simulink model "MWT_model"  (R2021b)
settings: Solver=VariableStepAuto  StartTime=0.0  StopTime=600  RelTol=1e-3
values from neighbouring files (symbols this model uses):
  Bt = 1e-6    (= 1e-06)    [MWT_model_input.m]
  Jt = 13.6e-7+1e-4    (= 0.00010136)    [MWT_model_input.m]
  Ke = Kt    (= 0.0139)    [MWT_model_input.m]
  Kt = 13.9e-3    (= 0.0139)    [MWT_model_input.m]
  La = 0.227    [MWT_model_input.m]
  p = 1.225    [MWT_model_input.m]
  p00 = 0.06736    [MWT_model_input.m]
  p01 = 0.279    [MWT_model_input.m]
  p02 = -0.09197    [MWT_model_input.m]
  p03 = 0.006537    [MWT_model_input.m]
  p10 = -0.01231    [MWT_model_input.m]
  p11 = 0.003341    [MWT_model_input.m]
  p12 = 0.002017    [MWT_model_input.m]
  p13 = -0.0001495    [MWT_model_input.m]
  p20 = 0.0001297    [MWT_model_input.m]
  p21 = -3.639e-05    [MWT_model_input.m]
  p22 = -1.063e-06    [MWT_model_input.m]
  p23 = 2.226e-07    [MWT_model_input.m]
  p30 = -4.46e-07    [MWT_model_input.m]
  p31 = 7.744e-08    [MWT_model_input.m]
  p32 = -1.905e-09    [MWT_model_input.m]
  p40 = 6.032e-10    [MWT_model_input.m]
  p41 = -4.972e-11    [MWT_model_input.m]
  p50 = -2.734e-13    [MWT_model_input.m]
  R = 0.75    [MWT_model_input.m]
  Ra = 2.07    [MWT_model_input.m]
  Vm = 3    [MWT_model_input.m]
  wcmax = 700    [MWT_model_input.m]
undefined symbols (not defined in the file or in its folder): sigbuilder_block
libraries: RCTblocks x2, simulink x1, slpidlib x1, autolibsharedcoupling x1
settings Model: Creator=alevl  LastModifiedBy=alevl

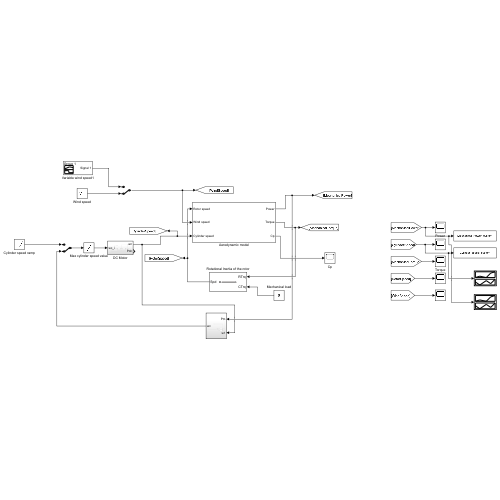
[thumbnail: Simulink's stored preview of the top-level diagram]
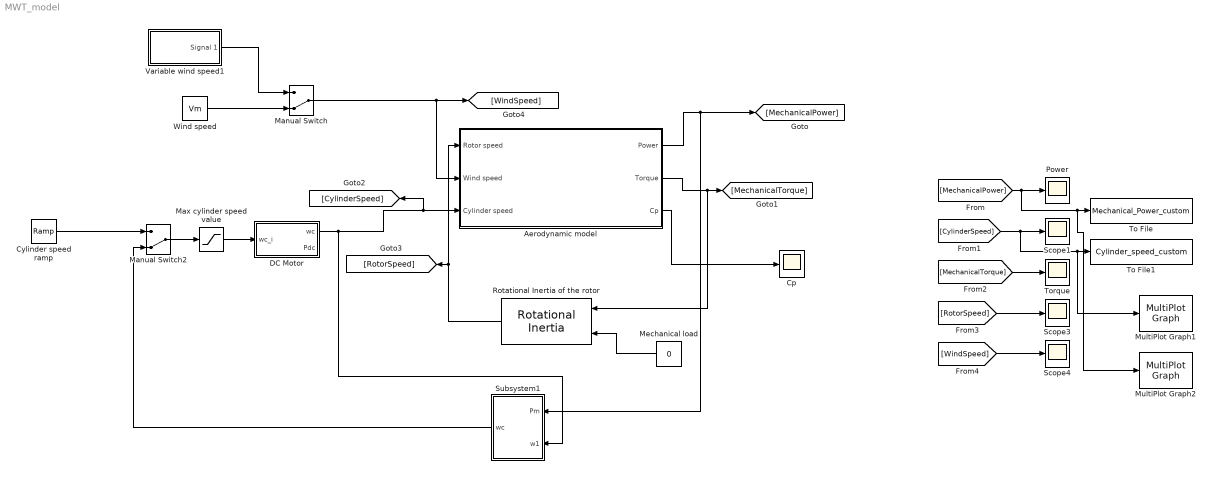
== system MWT_model ==
  Aerodynamic model : Subsystem
  Cp : Scope
  Cylinder speed ramp : simulink/Sources/Ramp  slope=1  start=0  InitialOutput=0
  DC Motor : Subsystem
  Manual Switch : ManualSwitch  CurrentSetting=0
  Manual Switch2 : ManualSwitch  CurrentSetting=0
  Max cylinder speed value : Saturate  UpperLimit=wcmax
  Mechanical load : Constant  Value=0
  MultiPlot Graph1 : RCTblocks/MultiPlot Graph  Tag=MultiPlot  tmin=0  tmax=350  ymin=0  ymax=700  Tsamp=-1  vnamesave=multisimout1
      settings: SourceProductBaseCode=RC
  MultiPlot Graph2 : RCTblocks/MultiPlot Graph  Tag=MultiPlot  tmin=0  tmax=350  ymin=0  ymax=600  Tsamp=-1  vnamesave=multisimout2
      settings: SourceProductBaseCode=RC
  Power : Scope
  Rotational Inertia of the rotor : autolibsharedcoupling/Rotational Inertia  port_config=Simulink  extInfo=off  externJ=off  J=2  b=1.4  omega_o=0.001  blkID=0  aMode=2
      settings: SourceProductBaseCode=PW,DR,MT,UV,VE
  Scope1 : Scope
  Scope3 : Scope
  Scope4 : Scope
  Subsystem1 : Subsystem
  To File : ToFile  Filename=Mechanical_Power_custom  MatrixName=P_NMPPT  SampleTime=0.01
  To File1 : ToFile  Filename=Cylinder_speed_custom  MatrixName=W_NMPPT  SampleTime=0.01
  Torque : Scope
  Variable wind speed1 : Subsystem  Tag=STV Subsys  LoadFcn=sigbuilder_block('load');  StartFcn=sigbuilder_block('start');  StopFcn=sigbuilder_block('stop');  ClipboardFcn=sigbuilder_block('clipboard');  mask(Sigbuilder block){tuvar=[0:10]}
      mask help: Simulink:masks:SigbuilderBlock_MD
      mask init:
      | if ~strcmp(get_param(bdroot(gcbh),'SimulationStatus'),'stopped') tuvar = sigbuilder_block('maskInit'); end
      settings: CopyFcn=sigbuilder_block('copy');  DeleteFcn=sigbuilder_block('delete');  ModelCloseFcn=sigbuilder_block('modelClose');  PreSaveFcn=sigbuilder_block('preSave');  PauseFcn=sigbuilder_block('pause');  ContinueFcn=sigbuilder_block('continue');  NameChangeFcn=sigbuilder_block('namechange');  OpenFcn=sigbuilder_block('open',[5.4 5.4 1141.2 580.8 ]);  CloseFcn=sigbuilder_block('close');
      mask Display: plot(0, 0, 100, 100,[2, 2, 32, 32, 2], [68, 8, 8, 68, 68],[32, 2], [38, 38], [32, 19, 2],[53, 60, 44], [32, 17, 17, 2],[16, 16, 31, 31]);txt = getActiveGroup(gcbh);text(2, 100, txt,'verticalAlignment', 'top');
  Wind speed : Constant  Value=Vm
  wires:
  Aerodynamic model/2(Torque) -> Rotational Inertia of the rotor/1, [MechanicalTorque]
  Rotational Inertia of the rotor/1 -> [RotorSpeed], Aerodynamic model/1(Rotor speed)
  Wind speed/1 -> Manual Switch/2
  Variable wind speed1/1(Signal 1) -> Manual Switch/1
  Manual Switch/1 -> Aerodynamic model/2(Wind speed), [WindSpeed]
  Cylinder speed ramp/1 -> Manual Switch2/1
  [MechanicalPower] -> MultiPlot Graph2/1, To File/1, Power/1
  [CylinderSpeed] -> MultiPlot Graph1/1, To File1/1, Scope1/1
  [MechanicalTorque] -> Torque/1
  [RotorSpeed] -> Scope3/1
  [WindSpeed] -> Scope4/1
  Aerodynamic model/1(Power) -> Subsystem1/1(Pm), [MechanicalPower]
  Aerodynamic model/3(Cp) -> Cp/1
  Mechanical load/1 -> Rotational Inertia of the rotor/2
  Manual Switch2/1 -> Max cylinder speed value/1
  Max cylinder speed value/1 -> DC Motor/1(wc_i)
  DC Motor/1(wc) -> Subsystem1/2(w1), Aerodynamic model/3(Cylinder speed), [CylinderSpeed]
  Subsystem1/1(wc) -> Manual Switch2/2

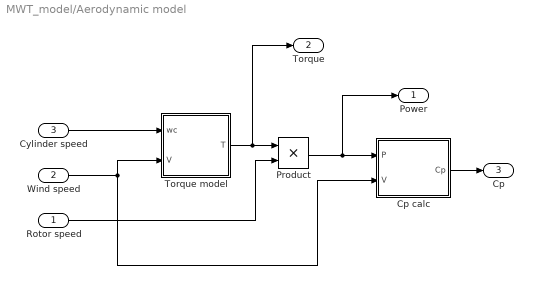
== system MWT_model/Aerodynamic model ==
  Rotor speed : Inport
  Wind speed : Inport  Port=2
  Cylinder speed : Inport  Port=3
  Cp calc : MATLAB Function  TreatAsAtomicUnit=on
  Product : Product
  Torque model : MATLAB Function  TreatAsAtomicUnit=on
  Power : Outport
  Torque : Outport  Port=2
  Cp : Outport  Port=3
  wires:
  Cylinder speed/1 -> Torque model/1(wc)
  Wind speed/1 -> Cp calc/2(V), Torque model/2(V)
  Torque model/1(T) -> Torque/1, Product/1
  Rotor speed/1 -> Product/2
  Product/1 -> Power/1, Cp calc/1(P)
  Cp calc/1(Cp) -> Cp/1

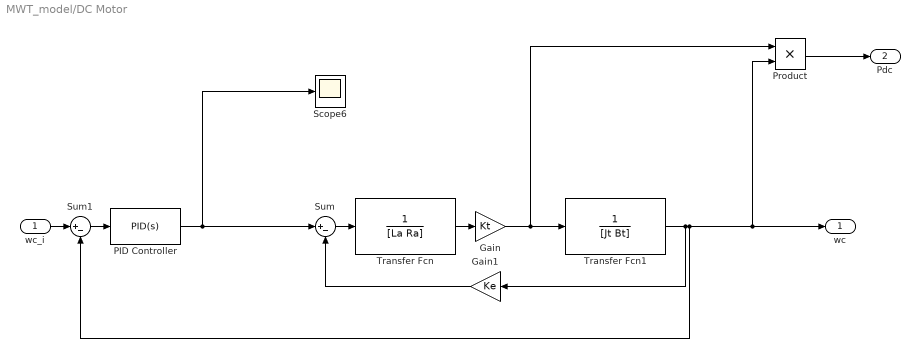
== system MWT_model/DC Motor ==
  wc_i : Inport
  Gain : Gain  Gain=Kt
  Gain1 : Gain  Gain=Ke
  PID Controller : slpidlib/PID Controller  Controller=PID  Form=Parallel  TimeDomain=Continuous-time  UseExternalTs=off  SampleTime=-1  IntegratorMethod=Forward Euler  FilterMethod=Forward Euler  ControllerParametersSource=internal  P=0.272229131767828  I=0.561292736049152  D=0.0312749136462088  UseFilter=on  N=2096.81611582006  TunerSelectOption=Transfer Function Based (PID Tuner App)  InitialConditionSource=internal  InitialConditionForIntegrator=0  InitialConditionForFilter=0  DifferentiatorICPrevScaledInput=0  ExternalReset=none  TrackingMode=off  Kt=1  LimitOutput=on  SatLimitsSource=internal  UpperSaturationLimit=12  LowerSaturationLimit=-12  LinearizeAsGain=on  AntiWindupMode=none  Kb=1  POutMin=[]  POutMax=[]  IOutMin=[]  IOutMax=[]  DOutMin=[]  DOutMax=[]  NOutMin=[]  NOutMax=[]  SumOutMin=[]  SumOutMax=[]  SaturationOutMin=[]  SaturationOutMax=[]  PParamMin=[]  PParamMax=[]  IParamMin=[]  IParamMax=[]  DParamMin=[]  DParamMax=[]  NParamMin=[]  NParamMax=[]  KbParamMin=[]  KbParamMax=[]  KtParamMin=[]  KtParamMax=[]  KbOutMin=[]  KbOutMax=[]  KtOutMin=[]  KtOutMax=[]  IntegratorOutMin=[]  IntegratorOutMax=[]  FilterOutMin=[]  FilterOutMax=[]  SumI1OutMin=[]  SumI1OutMax=[]  SumI2OutMin=[]  SumI2OutMax=[]  SumI3OutMin=[]  SumI3OutMax=[]  SumI4OutMin=[]  SumI4OutMax=[]  SumDOutMin=[]  SumDOutMax=[]  DifferentiatorOutMin=[]  DifferentiatorOutMax=[]  FilterDiffOutCoefMin=[]  FilterDiffOutCoefMax=[]  ReciprocalOutMin=[]  ReciprocalOutMax=[]  SumDenOutMin=[]  SumDenOutMax=[]  SumNumOutMin=[]  SumNumOutMax=[]  DivideOutMin=[]  DivideOutMax=[]  UdiffTsProdOutMin=[]  UdiffTsProdOutMax=[]  NTsProdOutMin=[]  NTsProdOutMax=[]  UintegralTsProdOutMin=[]  UintegralTsProdOutMax=[]  UngainTsProdOutMin=[]  UngainTsProdOutMax=[]  IntegratorContinuousStateAttributes=''  IntegratorStateMustResolveToSignalObject=off  IntegratorRTWStateStorageClass=Auto  FilterContinuousStateAttributes=''  FilterStateMustResolveToSignalObject=off  FilterRTWStateStorageClass=Auto  ParallelPVariant=InternalParameters  IdealPVariant=Disabled  IVariant=InternalParameters  DVariant=InternalParameters  IntegratorVariant=Continuous  SatVariant=Enabled  AWVariant=Passthrough  PCopyVariant=Disabled  TRVariant=Disabled  FdbkBlocksVariant=Forward  IdealPFdbkVariant=Disabled  SatFdbkVariant=Disabled  DerivativeFilterVariant=ContFilter  NVariant=InternalParameters  NCopyVariant=Disabled  FilterICVariant=InternalICsFilter  IntegratorICVariant=InternalICs  ExternalResetVariant=Disabled  TRSumVariant=Passthrough  SumFdbkVariant=Disabled  SumVariant=Sum_PID  TsampFilterVariant=InternalTs  TsampNgainVariant=Passthrough  TsampIntegralVariant=Passthrough  ExternalSaturationOutDataTypeStr=Inherit: Same as second input
  Product : Product
  Scope6 : Scope
  Sum : Sum  Inputs=|+-
  Sum1 : Sum  Inputs=|+-
  Transfer Fcn : TransferFcn  Denominator=[La Ra]
  Transfer Fcn1 : TransferFcn  Denominator=[Jt Bt]
  wc : Outport
  Pdc : Outport  Port=2
  wires:
  Transfer Fcn1/1 -> Product/2, wc/1, Sum1/2, Gain1/1
  wc_i/1 -> Sum1/1
  Sum1/1 -> PID Controller/1
  Gain1/1 -> Sum/2
  Sum/1 -> Transfer Fcn/1
  Product/1 -> Pdc/1
  Transfer Fcn/1 -> Gain/1
  PID Controller/1 -> Sum/1, Scope6/1
  Gain/1 -> Product/1, Transfer Fcn1/1

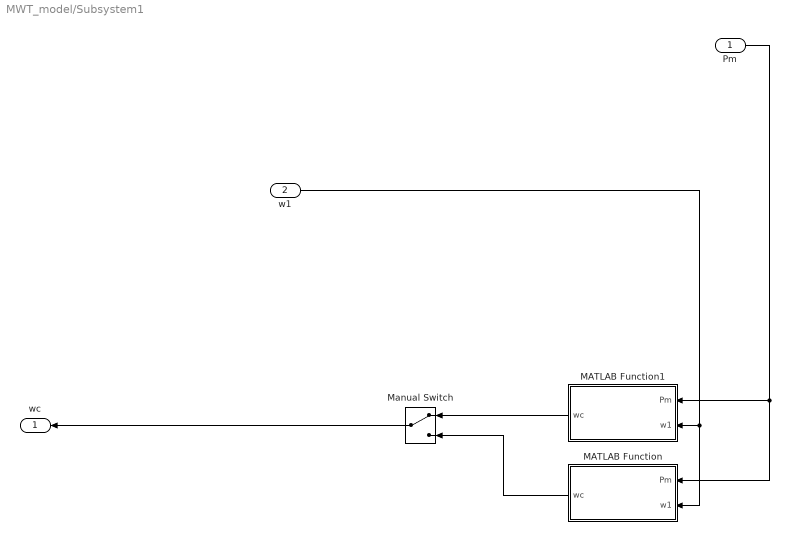
== system MWT_model/Subsystem1 ==
  Pm : Inport
  w1 : Inport  Port=2
  MATLAB Function : MATLAB Function  TreatAsAtomicUnit=on  SystemSampleTime=1
  MATLAB Function1 : MATLAB Function  TreatAsAtomicUnit=on  SystemSampleTime=1
  Manual Switch : ManualSwitch
  wc : Outport
  wires:
  MATLAB Function/1(wc) -> Manual Switch/2
  Pm/1 -> MATLAB Function/1(Pm), MATLAB Function1/1(Pm)
  w1/1 -> MATLAB Function/2(w1), MATLAB Function1/2(w1)
  MATLAB Function1/1(wc) -> Manual Switch/1
  Manual Switch/1 -> wc/1

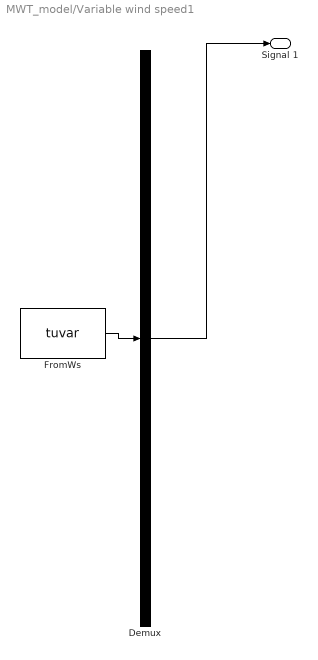
== system MWT_model/Variable wind speed1 ==
  Demux : Demux  Tag=STV Demux  Outputs=1
      settings: DisplayOption=none
  FromWs : FromWorkspace  Tag=STV FromWs  VariableName=tuvar
      SigBuilderData=|
      | common.afterFinalStr = 'Extrapolate'
      | common.sampleTime = 0
      | dataSet.timeRange = [0 350]
      | dataSet.name = 'Group 1'
      | sbobj.Groups.Name = 'Group 1'
      | sbobj.Groups.Signals.Name = 'Signal 1'
      | sbobj.Groups.Signals.XData = [0 50 50 100 100 150 150 200 200 250 250 300 300 350]
      | sbobj.Groups.Signals.YData = [2.5 2.5 5 5 7.5 7.5 10 10 7.5 7.5 5 5 2.5 2.5]
      | sbobj.Groups.TimeRange = [0 350]
  Signal 1 : Outport  Tag=STV Outport
  wires:
  FromWs/1 -> Demux/1
  Demux/1 -> Signal 1/1

== matlab function MWT_model/Subsystem1/MATLAB Function ==
  data: Pm input; wc output; w1 input
function wc = MPPT(Pm,w1)

%задание величин скорости вращения и мощности последовательными
persistent Pold wcold

%Задание начальных значений скорости вращения и мощности на первом шаге
if isempty (wcold)
    Pold=0;
    wcold=0;
end

%задание параметров алгоритма
wstep=30;

%цикл увеличения/уменьшения параметра исходя из состояния системы
if (Pm-Pold)>=0
    if (w1-wcold)>=0
        wc=w1+wstep;
    else
        wc=w1-wstep;
    end
else
    if (w1-wcold)>=0
        wc=w1-wstep;
    else
        wc=w1+wstep;
    end
end
%обвновление значений параметров по окончании цикла
wcold=w1;
Pold=Pm;

== matlab function MWT_model/Subsystem1/MATLAB Function1 ==
  data: Pm input; wc output; w1 input
function wc = HS_MPPT(Pm,w1)

%задание величин скорости вращения и мощности последовательными
persistent Pold wcold wstep i j EP
%Задание начальных значений скорости вращения и мощности на первом шаге
if isempty (wcold)
    Pold=0;
    wcold=0;
    wstep=30;
    i=0;
    j=0;
    EP=0;
end

%задание параметров алгоритма

EP=abs((Pold-Pm)/Pold)*100;
%цикл увеличения/уменьшения параметра исходя из состояния системы

if (Pm-Pold)>=0
    if (w1-wcold)>=0
        wc=w1+wstep;
    else
        wc=w1-wstep;
    end
else
    if (w1-wcold)>=0
        wc=w1-wstep;
    else
        wc=w1+wstep;
        wstep=wstep/2;
    end
end

% if (EP>0)&&(EP<=0.1)
%     wc=w1;
%     i=i+1;
% end

% if (i>2)&&(EP>0.1)
%     wstep=30;
%     i=0;
% end

if (EP>5)
    wstep=30;
    i=0;
end




if (wstep>30)
    wstep=30;
end


%обвновление значений параметров по окончании цикла
wcold=w1;
Pold=Pm;

== matlab function MWT_model/Aerodynamic model/Cp calc ==
  data: P input; Cp output; R parameter; p parameter; V input
function Cp= fcn(P,R, p, V)

A=pi*R^2;
Cp = P/(1/2*p*A*V^3);

== matlab function MWT_model/Aerodynamic model/Torque model ==
  data: wc input; T output; V input; p00 parameter; p10 parameter; p01 parameter; p20 parameter; p11 parameter; p02 parameter; p30 parameter; p21 parameter; p12 parameter; p03 parameter; p40 parameter; p31 parameter; p22 parameter; p13 parameter; p50 parameter; p41 parameter; p32 parameter; p23 parameter
function T = fcn(wc, V, p00, p10, p01, p20, p11, p02, p30, p21, p12, p03, p40, p31, p22, p13, p50, p41, p32, p23)
T = p00 + p10*wc + p01*V + p20*wc^2 + p11*wc*V + p02*V^2 + p30*wc^3 + p21*wc^2*V + p12*wc*V^2 + p03*V^3 + p40*wc^4 + p31*wc^3*V + p22*wc^2*V^2 + p13*wc*V^3 + p50*wc^5 + p41*wc^4*V + p32*wc^3*V^2 + p23*wc^2*V^3;
